simulink model "BasicRobotV3Animation"  (R2023b)
settings: Solver=VariableStepAuto  StartTime=0.0  StopTime=50.0  RelTol=1e-3
values from neighbouring files (symbols this model uses):
  floorsize = 50    [BasicRobot_Parameters.m]
  k_drag = 30    [BasicRobot_Parameters.m]
  m = 2.5    [BasicRobot_Parameters.m]
  r = 0.15    [BasicRobot_Parameters.m]
  r_ref = [3;4]    [BasicRobot_Parameters.m]
  rr_collide = 0.05    [BasicRobot_Parameters.m]
  rr_stop = 0.21    [BasicRobot_Parameters.m]
  rr_stop_dest = 0.16    [BasicRobot_Parameters.m]
  theta0 = deg2rad(theta0_deg)    [BasicRobot_Parameters.m]
  theta_ref = 1.50    (= 1.5)    [BasicRobot_Parameters.m]
  v_ref = 0.18    [BasicRobot_Parameters.m]
  x_obs = 0    [BasicRobot_Parameters.m]
  y_obs = 0    [BasicRobot_Parameters.m]
undefined symbols (not defined in the file or in its folder): magnitude
libraries: simulink x7, vrlib x2
settings Model: Creator=BeanieBabyJ  LastModifiedBy=BeanieBabyJ
settings SolverCC: ZeroCrossAlgorithm=Adaptive
settings DebuggingCC: IgnoredZcDiagnostic=none

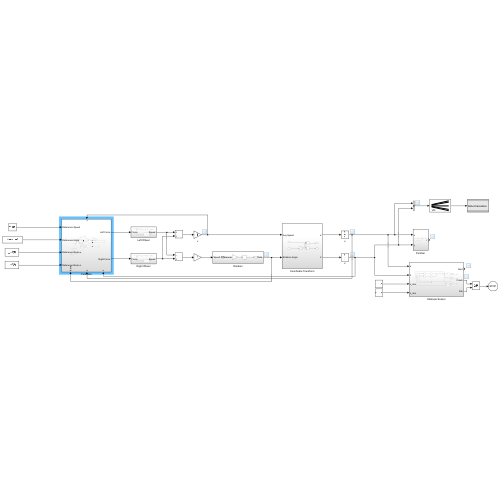
[thumbnail: Simulink's stored preview of the top-level diagram]
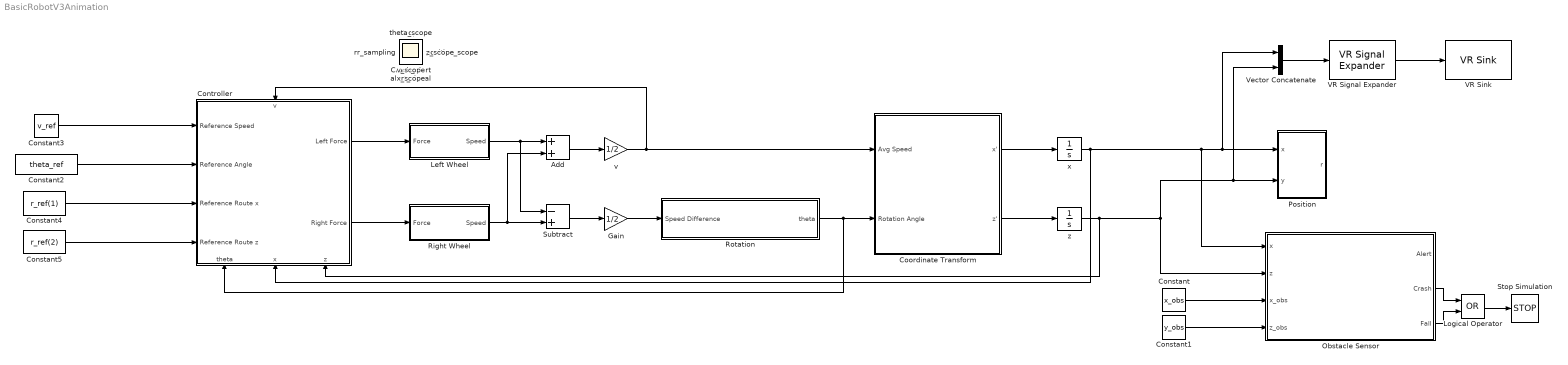
== system BasicRobotV3Animation ==
  Add : Sum
  Constant : Constant  Value=x_obs
  Constant1 : Constant  Value=y_obs
  Constant2 : Constant  Value=theta_ref
  Constant3 : Constant  Value=v_ref
  Constant4 : Constant  Value=r_ref(1)
  Constant5 : Constant  Value=r_ref(2)
  Controller : Subsystem
      settings: PortSchema="{\"entries\":[{\"content\":{\"sides\":[{\"content\":{\"connectorIds\":[\"In1\",\"In2\",\"In3\",\"In4\"]},\"type\":\"ConnectorPlacement.EquallySpacedRectSide\",\"uuid\":\"ba94545e-9c5b-44f0-b142-601db8af74fa\"},{\"content\":{\"connectorIds\":[\"Out1\",\"Out2\"],\"side\":\"RIGHT\"},\"type\":\"ConnectorPlacement.EquallySpacedRectSide\",\"uuid\":\"af029479-1ae4-4d42-872b-d9816a1308e5\"},{\"content\":{\"connectorIds\":[\"In5\"],\"side\":\"TOP\"},\"type\":\"ConnectorPlacement.EquallySpacedRectSide\",\"uuid\":\"a7d99619-4318-4ae9-a369-f3fafeea2edf\"},{\"content\":{\"connectorIds\":[\"In6\",\"In7\",\"In8\"],\"side\":\"BOTTOM\"},\"type\":\"ConnectorPlacement.EquallySpacedRectSide\",\"uuid\":\"9d977537-dbbb-45bb-88a3-801d5ac276a0\"}]},\"type\":\"ConnectorPlacement.EquallySpacedConnector\",\"uuid\":\"d5be0c1c-28be-41e4-a0b4-1100c8fad692\"}],\"packageUris\":[\"http://schema.mathworks.com/mf0/Connector/R2020b\"],\"version\":\"1.0\"}"
  Coordinate Transform : Subsystem
  Gain : Gain  Gain=1/2
  Left Wheel : Subsystem
  Logical Operator : Logic  Operator=OR  AllPortsSameDT=off  OutDataTypeStr=boolean
  Obstacle Sensor : Subsystem
  Position : Subsystem
  Right Wheel : Subsystem
  Rotation : Subsystem
  Stop Simulation : Stop
  Subtract : Sum  Inputs=-+
  VR Signal Expander : vrlib/VR Signal Expander  outwidth=3  outidx=[1 3]
  VR Sink : vrlib/VR Sink  InstantiateOnLoad=on  SampleTime=0.1  ViewEnable=on  RemoteChange=off  RemoteView=off  FieldsWritten=Robot.translation.3.1.1.double  WorldFileName=RobotWorld.wrl  AutoView=off  VideoDimensions=[]  AllowVariableSize=off
  Vector Concatenate : Concatenate
  v : Gain  Gain=1/2
  x : Integrator
  z : Integrator
  Crash_alert : Scope
  Scope : Scope
  alert_signal : Scope
  position_scope : Scope
  rr_sampling : Scope
  theta_scope : Scope
  v_scope : Scope
  x_scope : Scope
  z_scope : Scope
  wires:
  Right Wheel/1(Speed) -> Add/2, Subtract/2
  Left Wheel/1(Speed) -> Add/1, Subtract/1
  Subtract/1 -> Gain/1
  Gain/1 -> Rotation/1(Speed Difference)
  Add/1 -> v/1
  v/1 -> Coordinate Transform/1(Avg Speed), Controller/5(v)
  Controller/2(Right Force) -> Right Wheel/1(Force)
  Coordinate Transform/1(x') -> x/1
  Coordinate Transform/2(z') -> z/1
  Controller/1(Left Force) -> Left Wheel/1(Force)
  x/1 -> Vector Concatenate/1, Position/1(x), Obstacle Sensor/1(x), Controller/7(x)
  z/1 -> Vector Concatenate/2, Position/2(y), Obstacle Sensor/2(z), Controller/8(z)
  Constant/1 -> Obstacle Sensor/3(x_obs)
  Constant1/1 -> Obstacle Sensor/4(z_obs)
  Rotation/1(theta) -> Controller/6(theta), Coordinate Transform/2(Rotation Angle)
  VR Signal Expander/1 -> VR Sink/1
  Vector Concatenate/1 -> VR Signal Expander/1
  Obstacle Sensor/2(Crash) -> Logical Operator/1
  Obstacle Sensor/3(Fall) -> Logical Operator/2
  Logical Operator/1 -> Stop Simulation/1
  Constant3/1 -> Controller/1(Reference Speed)
  Constant2/1 -> Controller/2(Reference Angle)
  Constant4/1 -> Controller/3(Reference Route x)
  Constant5/1 -> Controller/4(Reference Route z)

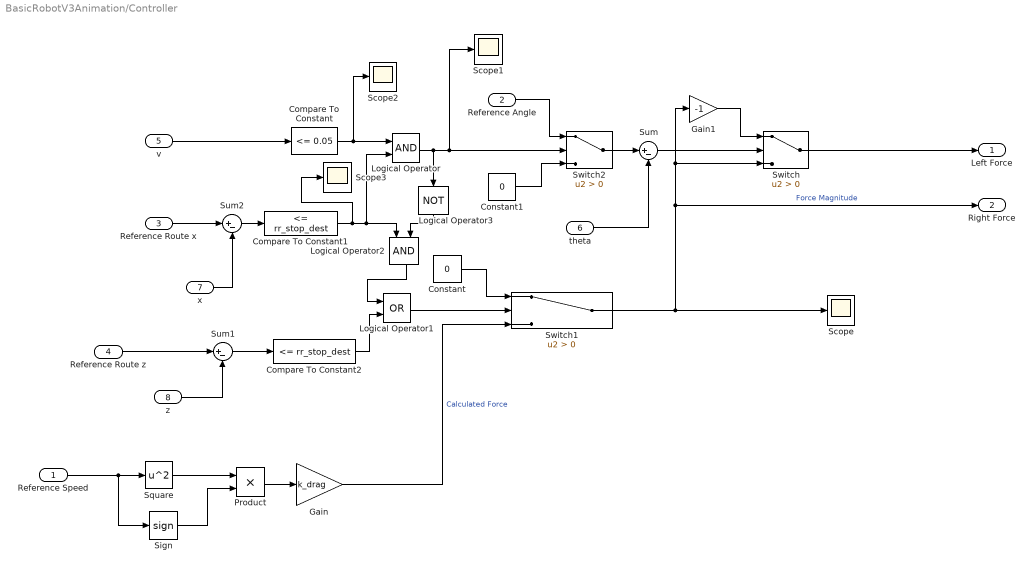
== system BasicRobotV3Animation/Controller ==
  Reference Speed : Inport
  Reference Angle : Inport  Port=2
  Reference Route x : Inport  Port=3
  Reference Route z : Inport  Port=4
  v : Inport  Port=5
  theta : Inport  Port=6
  x : Inport  Port=7
  z : Inport  Port=8
  Compare To Constant : simulink/Logic and Bit Operations/Compare To Constant  relop=<=  const=0.05  OutDataTypeStr=boolean
  Compare To Constant1 : simulink/Logic and Bit Operations/Compare To Constant  relop=<=  const=rr_stop_dest  OutDataTypeStr=boolean
  Compare To Constant2 : simulink/Logic and Bit Operations/Compare To Constant  relop=<=  const=rr_stop_dest  OutDataTypeStr=boolean
  Constant : Constant  Value=0
  Constant1 : Constant  Value=0
  Gain : Gain  Gain=k_drag
  Gain1 : Gain  Gain=-1
  Logical Operator : Logic  AllPortsSameDT=off  OutDataTypeStr=boolean
  Logical Operator1 : Logic  Operator=OR  AllPortsSameDT=off  OutDataTypeStr=boolean
  Logical Operator2 : Logic  AllPortsSameDT=off  OutDataTypeStr=boolean
  Logical Operator3 : Logic  Operator=NOT  AllPortsSameDT=off  OutDataTypeStr=boolean
  Product : Product
  Scope{,1..3} (4 alike) : Scope
  Sign : Signum
  Square : Math  Operator=square
  Sum : Sum  Inputs=|+-
  Sum1 : Sum  Inputs=|+-
  Sum2 : Sum  Inputs=|+-
  Switch : Switch  Criteria=u2 > Threshold  SaturateOnIntegerOverflow=off  InputSameDT=off
  Switch1 : Switch  Criteria=u2 > Threshold  SaturateOnIntegerOverflow=off  InputSameDT=off
  Switch2 : Switch  Criteria=u2 > Threshold  SaturateOnIntegerOverflow=off  InputSameDT=off
  Left Force : Outport
  Right Force : Outport  Port=2
  wires:
  theta/1 -> Sum/2
  Sum/1 -> Switch/2
  Switch/1 -> Left Force/1
  Gain1/1 -> Switch/1
  Reference Speed/1 -> Sign/1, Square/1
  Square/1 -> Product/1
  Sign/1 -> Product/2
  Product/1 -> Gain/1
  Gain/1 -> Switch1/3  "Calculated Force"
  Switch1/1 -> Scope/1, Right Force/1, Switch/3, Gain1/1  "Force Magnitude"
  Constant/1 -> Switch1/1
  Switch2/1 -> Sum/1
  v/1 -> Compare To Constant/1
  Compare To Constant/1 -> Scope2/1, Logical Operator/1
  Constant1/1 -> Switch2/3
  Reference Angle/1 -> Switch2/1
  Reference Route x/1 -> Sum2/1
  Reference Route z/1 -> Sum1/1
  Sum2/1 -> Compare To Constant1/1
  Compare To Constant1/1 -> Scope3/1, Logical Operator/2, Logical Operator2/1
  Sum1/1 -> Compare To Constant2/1
  x/1 -> Sum2/2
  z/1 -> Sum1/2
  Logical Operator1/1 -> Switch1/2
  Compare To Constant2/1 -> Logical Operator1/2
  Logical Operator2/1 -> Logical Operator1/1
  Logical Operator3/1 -> Logical Operator2/2
  Logical Operator/1 -> Logical Operator3/1, Scope1/1, Switch2/2

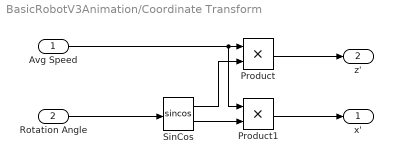
== system BasicRobotV3Animation/Coordinate Transform ==
  Avg Speed : Inport
  Rotation Angle : Inport  Port=2
  Product : Product
  Product1 : Product
  SinCos : Trigonometry  Operator=sincos
  x' : Outport
  z' : Outport  Port=2
  wires:
  Rotation Angle/1 -> SinCos/1
  Avg Speed/1 -> Product1/1, Product/1
  SinCos/1 -> Product/2
  SinCos/2 -> Product1/2
  Product/1 -> z'/1
  Product1/1 -> x'/1

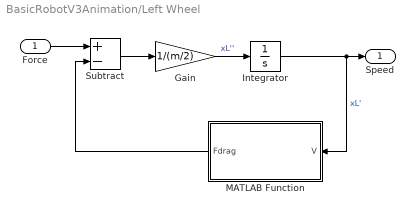
== system BasicRobotV3Animation/Left Wheel ==
  Force : Inport
  Gain : Gain  Gain=1/(m/2)
  Integrator : Integrator
  MATLAB Function : MATLAB Function  TreatAsAtomicUnit=on
  Subtract : Sum  Inputs=+-
  Speed : Outport
  wires:
  Force/1 -> Subtract/1
  MATLAB Function/1(Fdrag) -> Subtract/2
  Subtract/1 -> Gain/1
  Integrator/1 -> MATLAB Function/1(V), Speed/1  "xL'"
  Gain/1 -> Integrator/1  "xL''"

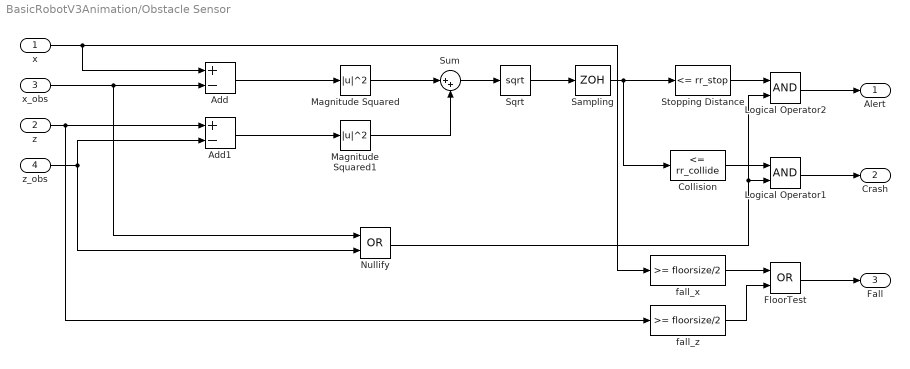
== system BasicRobotV3Animation/Obstacle Sensor ==
  x : Inport
  z : Inport  Port=2
  x_obs : Inport  Port=3
  z_obs : Inport  Port=4
  Add : Sum  Inputs=+-
  Add1 : Sum  Inputs=+-
  Collision : simulink/Logic and Bit Operations/Compare To Constant  relop=<=  const=rr_collide  OutDataTypeStr=boolean
  FloorTest : Logic  Operator=OR  AllPortsSameDT=off  OutDataTypeStr=boolean
  Logical Operator1 : Logic  AllPortsSameDT=off  OutDataTypeStr=boolean
  Logical Operator2 : Logic  AllPortsSameDT=off  OutDataTypeStr=boolean
  Magnitude Squared : Math  Operator=magnitude^2
  Magnitude Squared1 : Math  Operator=magnitude^2
  Nullify : Logic  Operator=OR  AllPortsSameDT=off  OutDataTypeStr=boolean
  Sampling : ZeroOrderHold  SampleTime=0.25
  Sqrt : Sqrt
  Stopping Distance : simulink/Logic and Bit Operations/Compare To Constant  relop=<=  const=rr_stop  OutDataTypeStr=boolean
  Sum : Sum  Inputs=|++
  fall_x : simulink/Logic and Bit Operations/Compare To Constant  relop=>=  const=floorsize/2  OutDataTypeStr=boolean
  fall_z : simulink/Logic and Bit Operations/Compare To Constant  relop=>=  const=floorsize/2  OutDataTypeStr=boolean
  Alert : Outport
  Crash : Outport  Port=2
  Fall : Outport  Port=3
  wires:
  Sampling/1 -> Collision/1, Stopping Distance/1
  x/1 -> fall_x/1, Add/1
  Magnitude Squared/1 -> Sum/1
  Sum/1 -> Sqrt/1
  Add/1 -> Magnitude Squared/1
  Add1/1 -> Magnitude Squared1/1
  Sqrt/1 -> Sampling/1
  x_obs/1 -> Nullify/1, Add/2
  z/1 -> fall_z/1, Add1/1
  z_obs/1 -> Nullify/2, Add1/2
  Magnitude Squared1/1 -> Sum/2
  Collision/1 -> Logical Operator1/1
  Logical Operator1/1 -> Crash/1
  Nullify/1 -> Logical Operator2/2, Logical Operator1/2
  Stopping Distance/1 -> Logical Operator2/1
  Logical Operator2/1 -> Alert/1
  fall_x/1 -> FloorTest/1
  FloorTest/1 -> Fall/1
  fall_z/1 -> FloorTest/2

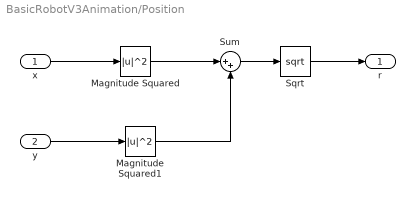
== system BasicRobotV3Animation/Position ==
  x : Inport
  y : Inport  Port=2
  Magnitude Squared : Math  Operator=magnitude^2
  Magnitude Squared1 : Math  Operator=magnitude^2
  Sqrt : Sqrt
  Sum : Sum  Inputs=|++
  r : Outport
  wires:
  Magnitude Squared1/1 -> Sum/2
  Sum/1 -> Sqrt/1
  Magnitude Squared/1 -> Sum/1
  Sqrt/1 -> r/1
  x/1 -> Magnitude Squared/1
  y/1 -> Magnitude Squared1/1

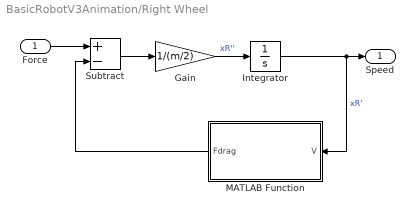
== system BasicRobotV3Animation/Right Wheel ==
  Force : Inport
  Gain : Gain  Gain=1/(m/2)
  Integrator : Integrator
  MATLAB Function : MATLAB Function  TreatAsAtomicUnit=on
  Subtract : Sum  Inputs=+-
  Speed : Outport
  wires:
  Integrator/1 -> MATLAB Function/1(V), Speed/1  "xR'"
  Gain/1 -> Integrator/1  "xR''"
  Force/1 -> Subtract/1
  MATLAB Function/1(Fdrag) -> Subtract/2
  Subtract/1 -> Gain/1

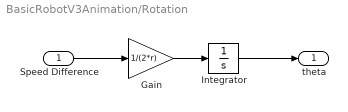
== system BasicRobotV3Animation/Rotation ==
  Speed Difference : Inport
  Gain : Gain  Gain=1/(2*r)
  Integrator : Integrator  InitialCondition=theta0
  theta : Outport
  wires:
  Speed Difference/1 -> Gain/1
  Gain/1 -> Integrator/1
  Integrator/1 -> theta/1

== matlab function BasicRobotV3Animation/Right Wheel/MATLAB Function ==
  data: Fdrag output; V input; k_drag parameter
function Fdrag=get_fdrag(V, k_drag)

Fdrag=k_drag*V*abs(V);

== matlab function BasicRobotV3Animation/Left Wheel/MATLAB Function ==
  data: Fdrag output; V input; k_drag parameter
function Fdrag=get_fdrag(V, k_drag)

Fdrag=k_drag*V*abs(V);
